simulink model "mrefrobotarm_modified_previous_y_previous_u_previous_ref_pert_2"  (R2018b)
settings: Solver=FixedStepAuto  StartTime=0.0  StopTime=60  RelTol=1e-3  AbsTol=1e-6
undefined symbols (not defined in the file or in its folder): cc, options
libraries: neural x858, simulink x1
(part 10 of 32)

== system mrefrobotarm_modified_previous_y_previous_u_previous_ref_pert_2/m=0 sd=0 original/Layer 3/Delays 1 ==
  "p{3}" : Inport  PortDimensions=30
      mask Display: e = 0.06;c1 = [120 230 180]/255;c2 = ([120 230 180]+0)/(256+128);c3 = ([120 230 180]+128)/(256+128);patch([0 1 1 0],[0 0 1 1],c1);patch([0 1 1 1-e 1-e 0+e],[0 0 1 1-e 0+e 0+e],c2);patch([0 0 1 1-e 0+e 0+e],[0 1 1 1-e 1-e 0+e],c3);plot([0 1 1 0 0],[0 0 1 1 0]);
  mux : Mux  Inputs=1
      mask Display: e = 0.06;c1 = [120 150 230]/255;c2 = ([120 150 230]+0)/383;c3 = ([120 150 230]+128)/383;patch([0 1 1 0],[0 0 1 1],c1);patch([0 1 1 1-e 1-e 0+e],[0 0 1 1-e 0+e 0+e],c2);patch([0 0 1 1-e 0+e 0+e],[0 1 1 1-e 1-e 0+e],c3);plot([0 1 1 0 0],[0 0 1 1 0]);disp('Mux')
  "pd{3,2}" : Outport
      mask Display: e = 0.06;c1 = [120 230 180]/255;c2 = ([120 230 180]+0)/(256+128);c3 = ([120 230 180]+128)/(256+128);patch([0 1 1 0],[0 0 1 1],c1);patch([0 1 1 1-e 1-e 0+e],[0 0 1 1-e 0+e 0+e],c2);patch([0 0 1 1-e 0+e 0+e],[0 1 1 1-e 1-e 0+e],c3);plot([0 1 1 0 0],[0 0 1 1 0]);
  wires:
  "p{3}"/1 -> mux/1
  mux/1 -> "pd{3,2}"/1

== system mrefrobotarm_modified_previous_y_previous_u_previous_ref_pert_2/m=0 sd=0 original/Layer 3/LW{3,2} ==
  "ad{3,2}" : Inport  PortDimensions=30
      mask Display: e = 0.06;c1 = [120 230 180]/255;c2 = ([120 230 180]+0)/(256+128);c3 = ([120 230 180]+128)/(256+128);patch([0 1 1 0],[0 0 1 1],c1);patch([0 1 1 1-e 1-e 0+e],[0 0 1 1-e 0+e 0+e],c2);patch([0 0 1 1-e 0+e 0+e],[0 1 1 1-e 1-e 0+e],c3);plot([0 1 1 0 0],[0 0 1 1 0]);
  "IW{3,2}(1,:)'" : Constant  Value=[0.17482246150930424999359047433244995772838592529296875;0.55622207112490962277462358542834408581256866455078125;0.0031372872160854207122804293561557642533443868160247802734375;-0.168108405397883908793943419368588365614414215087890625;0.05837691976433061202822472068874049000442028045654296875;-0.402959678570381563122992929493193514645099639892578125;-0.167155303188543158388057463525910861790180206298828125;-0.1338968343609756583845182831282727420330047607421875;0.14686670623474251673457047218107618391513824462890625;0.01157271158637744427888360831957470509223639965057373046875;-0.1531146663300509136451665881395456381142139434814453125;0.0190428533611202814579410613760046544484794139862060546875;-0.2039279411341271275315278899142867885529994964599609375;-0.003914288286597765627317091485792843741364777088165283203125;-0.2328617323239242919985514390646130777895450592041015625;0.1159952622429807345127983353449963033199310302734375;0.462684207486491916316850847579189576208591461181640625;-0.01074998441387134580360385172070891712792217731475830078125;-0.464908519270919862176327796987607143819332122802734375;0.098111452853946179430977281299419701099395751953125;0.00777207254254363121004356429466497502289712429046630859375;-0.1946466427188742187581738107837736606597900390625;0.01549753182636756827783575118928638403303921222686767578125;-0.0263655234629284855596420555912118288688361644744873046875;0.11790973762661406676333086807062500156462192535400390625;0.001769238327251491764424695674051690730266273021697998046875;-0.00594124961309642173057365965860299183987081050872802734375;-0.452866633892114067716505587668507359921932220458984375;-0.15777748494897725350938344490714371204376220703125;-0.57998766696437631384952737789717502892017364501953125]
      mask Display: e = 0.06;c1 = [120 150 230]/255;c2 = ([120 150 230]+0)/383;c3 = ([120 150 230]+128)/383;patch([0 1 1 0],[0 0 1 1],c1);patch([0 1 1 1-e 1-e 0+e],[0 0 1 1-e 0+e 0+e],c2);patch([0 0 1 1-e 0+e 0+e],[0 1 1 1-e 1-e 0+e],c3);plot([0 1 1 0 0],[0 0 1 1 0]);disp('weights');
  Mux : Mux  Inputs=1
      mask Display: e = 0.06;c1 = [120 150 230]/255;c2 = ([120 150 230]+0)/383;c3 = ([120 150 230]+128)/383;patch([0 1 1 0],[0 0 1 1],c1);patch([0 1 1 1-e 1-e 0+e],[0 0 1 1-e 0+e 0+e],c2);patch([0 0 1 1-e 0+e 0+e],[0 1 1 1-e 1-e 0+e],c3);plot([0 1 1 0 0],[0 0 1 1 0]);disp('Mux');
  dotprod1 : neural/Weight Functions/dotprod
  "lz{3,2}" : Outport
      mask Display: e = 0.06;c1 = [120 230 180]/255;c2 = ([120 230 180]+0)/(256+128);c3 = ([120 230 180]+128)/(256+128);patch([0 1 1 0],[0 0 1 1],c1);patch([0 1 1 1-e 1-e 0+e],[0 0 1 1-e 0+e 0+e],c2);patch([0 0 1 1-e 0+e 0+e],[0 1 1 1-e 1-e 0+e],c3);plot([0 1 1 0 0],[0 0 1 1 0]);
  wires:
  "IW{3,2}(1,:)'"/1 -> dotprod1/1
  "ad{3,2}"/1 -> dotprod1/2
  dotprod1/1 -> Mux/1
  Mux/1 -> "lz{3,2}"/1

== system mrefrobotarm_modified_previous_y_previous_u_previous_ref_pert_2/m=0 sd=0.001/Layer 1/Delays 1 ==
  "p{1}" : Inport  PortDimensions=10
      mask Display: e = 0.06;c1 = [120 230 180]/255;c2 = ([120 230 180]+0)/(256+128);c3 = ([120 230 180]+128)/(256+128);patch([0 1 1 0],[0 0 1 1],c1);patch([0 1 1 1-e 1-e 0+e],[0 0 1 1-e 0+e 0+e],c2);patch([0 0 1 1-e 0+e 0+e],[0 1 1 1-e 1-e 0+e],c3);plot([0 1 1 0 0],[0 0 1 1 0]);
  mux : Mux  Inputs=1
      mask Display: e = 0.06;c1 = [120 150 230]/255;c2 = ([120 150 230]+0)/383;c3 = ([120 150 230]+128)/383;patch([0 1 1 0],[0 0 1 1],c1);patch([0 1 1 1-e 1-e 0+e],[0 0 1 1-e 0+e 0+e],c2);patch([0 0 1 1-e 0+e 0+e],[0 1 1 1-e 1-e 0+e],c3);plot([0 1 1 0 0],[0 0 1 1 0]);disp('Mux')
  "pd{1,1}" : Outport
      mask Display: e = 0.06;c1 = [120 230 180]/255;c2 = ([120 230 180]+0)/(256+128);c3 = ([120 230 180]+128)/(256+128);patch([0 1 1 0],[0 0 1 1],c1);patch([0 1 1 1-e 1-e 0+e],[0 0 1 1-e 0+e 0+e],c2);patch([0 0 1 1-e 0+e 0+e],[0 1 1 1-e 1-e 0+e],c3);plot([0 1 1 0 0],[0 0 1 1 0]);
  wires:
  "p{1}"/1 -> mux/1
  mux/1 -> "pd{1,1}"/1

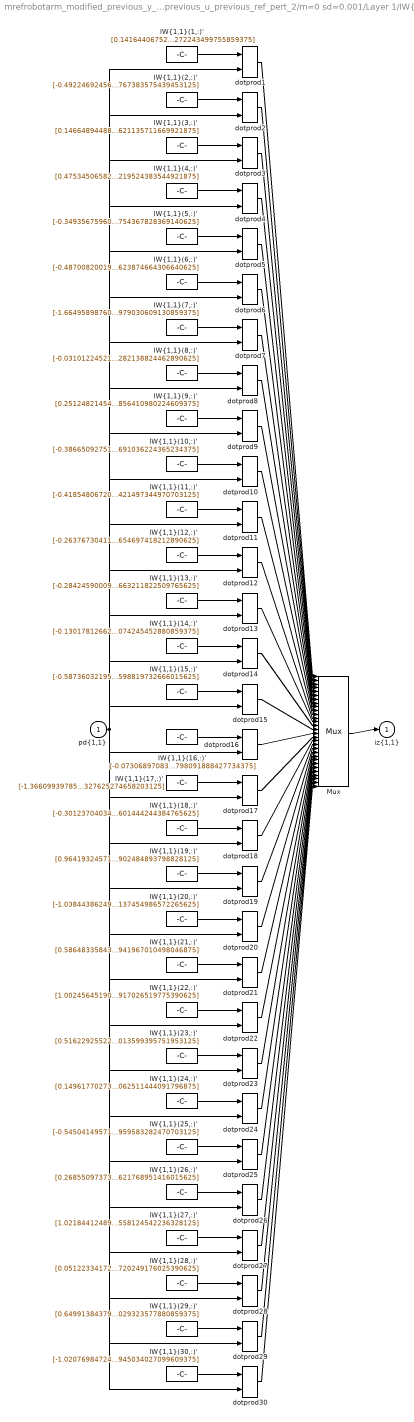
== system mrefrobotarm_modified_previous_y_previous_u_previous_ref_pert_2/m=0 sd=0.001/Layer 1/IW{1,1} ==
  "pd{1,1}" : Inport  PortDimensions=10
      mask Display: e = 0.06;c1 = [120 230 180]/255;c2 = ([120 230 180]+0)/(256+128);c3 = ([120 230 180]+128)/(256+128);patch([0 1 1 0],[0 0 1 1],c1);patch([0 1 1 1-e 1-e 0+e],[0 0 1 1-e 0+e 0+e],c2);patch([0 0 1 1-e 0+e 0+e],[0 1 1 1-e 1-e 0+e],c3);plot([0 1 1 0 0],[0 0 1 1 0]);
  "IW{1,1}(1,:)'" : Constant  Value=[0.141644067527063766132044975165626965463161468505859375;-0.040811020431186666168610344129774603061378002166748046875;-0.312974436634471164797588471628841944038867950439453125;0.04886853485988666701000937564458581618964672088623046875;-0.82641893263483934273239128742716275155544281005859375;-0.91587297277856272170737383930827490985393524169921875;0.67313210047715543726809528379817493259906768798828125;-0.039377277910727627452391885753968381322920322418212890625;-1.2808123988443942398163244433817453682422637939453125;-1.19270082118834519491201717755757272243499755859375]
      mask Display: e = 0.06;c1 = [120 150 230]/255;c2 = ([120 150 230]+0)/383;c3 = ([120 150 230]+128)/383;patch([0 1 1 0],[0 0 1 1],c1);patch([0 1 1 1-e 1-e 0+e],[0 0 1 1-e 0+e 0+e],c2);patch([0 0 1 1-e 0+e 0+e],[0 1 1 1-e 1-e 0+e],c3);plot([0 1 1 0 0],[0 0 1 1 0]);disp('Weights');
  "IW{1,1}(10,:)'" : Constant  Value=[-0.38665092751456509034824193804524838924407958984375;0.06410981472709277595445342967650503851473331451416015625;0.11657362993113169757908309520644252188503742218017578125;0.034769749880571333700007841116530471481382846832275390625;-0.2113731343708413479287600011957692913711071014404296875;1.3959509118760367041289782719104550778865814208984375;-1.3344611781825508334264895893284119665622711181640625;-0.26325521537912710545725758493063040077686309814453125;1.11568339513819214658951750607229769229888916015625;0.285147448344198417569117509628995321691036224365234375]
      mask Display: e = 0.06;c1 = [120 150 230]/255;c2 = ([120 150 230]+0)/383;c3 = ([120 150 230]+128)/383;patch([0 1 1 0],[0 0 1 1],c1);patch([0 1 1 1-e 1-e 0+e],[0 0 1 1-e 0+e 0+e],c2);patch([0 0 1 1-e 0+e 0+e],[0 1 1 1-e 1-e 0+e],c3);plot([0 1 1 0 0],[0 0 1 1 0]);disp('Weights');
  "IW{1,1}(11,:)'" : Constant  Value=[-0.4185480672053982775793201653868891298770904541015625;-0.1705980694049138157719625041863764636218547821044921875;-0.0190899797350324341993488275193158187903463840484619140625;-0.327569152910229366426619890262372791767120361328125;0.1274098816431911418423084114692755974829196929931640625;-1.9161340172549110594246712935273535549640655517578125;0.05443650875980780845520001776094431988894939422607421875;0.32968385223698126740288216751650907099246978759765625;-0.98609685726316964604620807222090661525726318359375;-1.012171418694518099101742336642928421497344970703125]
      mask Display: e = 0.06;c1 = [120 150 230]/255;c2 = ([120 150 230]+0)/383;c3 = ([120 150 230]+128)/383;patch([0 1 1 0],[0 0 1 1],c1);patch([0 1 1 1-e 1-e 0+e],[0 0 1 1-e 0+e 0+e],c2);patch([0 0 1 1-e 0+e 0+e],[0 1 1 1-e 1-e 0+e],c3);plot([0 1 1 0 0],[0 0 1 1 0]);disp('Weights');
  "IW{1,1}(12,:)'" : Constant  Value=[-0.263767304113963263478837006914545781910419464111328125;-0.629903348227637049916438627406023442745208740234375;0.7293914306477302655906669315299950540065765380859375;0.1405283307055230357374142613480216823518276214599609375;1.7781482645602564307552029276848770678043365478515625;-2.97153163801516040365413573454134166240692138671875;0.443336274156811371849329361793934367597103118896484375;0.55612212810498140580506287733442150056362152099609375;-0.1887978911441915153002213401123299263417720794677734375;-0.55133598654912996384069856503629125654697418212890625]
      mask Display: e = 0.06;c1 = [120 150 230]/255;c2 = ([120 150 230]+0)/383;c3 = ([120 150 230]+128)/383;patch([0 1 1 0],[0 0 1 1],c1);patch([0 1 1 1-e 1-e 0+e],[0 0 1 1-e 0+e 0+e],c2);patch([0 0 1 1-e 0+e 0+e],[0 1 1 1-e 1-e 0+e],c3);plot([0 1 1 0 0],[0 0 1 1 0]);disp('Weights');
  "IW{1,1}(13,:)'" : Constant  Value=[-0.2842459000975889882312230838579125702381134033203125;-0.07040272701257387077955485210623010061681270599365234375;-0.279039840893809010236026324491831474006175994873046875;-0.89305639600684505463590312501764856278896331787109375;3.341208886966132052265265883761458098888397216796875;-1.98213319967933188081588014028966426849365234375;-0.90166622936895013395997011684812605381011962890625;0.2060321618557637013413597060207393951714038848876953125;0.00677792762518984910624642026277797413058578968048095703125;0.7006967694845107619272539523080922663211822509765625]
      mask Display: e = 0.06;c1 = [120 150 230]/255;c2 = ([120 150 230]+0)/383;c3 = ([120 150 230]+128)/383;patch([0 1 1 0],[0 0 1 1],c1);patch([0 1 1 1-e 1-e 0+e],[0 0 1 1-e 0+e 0+e],c2);patch([0 0 1 1-e 0+e 0+e],[0 1 1 1-e 1-e 0+e],c3);plot([0 1 1 0 0],[0 0 1 1 0]);disp('Weights');
  "IW{1,1}(14,:)'" : Constant  Value=[-0.130178126624194090421582359340391121804714202880859375;-0.57366570129351235340919856753316707909107208251953125;0.339047467618743325612484795783529989421367645263671875;0.09356817756562685328702855258597992360591888427734375;-2.342341044490604762273733285837806761264801025390625;0.73263251994819456047736139225889928638935089111328125;-1.0945043994785914609479959835880436003208160400390625;0.36014660154459676721927507969667203724384307861328125;0.08590539675617943349283933685001102276146411895751953125;0.294060428112707439307627055313787423074245452880859375]
      mask Display: e = 0.06;c1 = [120 150 230]/255;c2 = ([120 150 230]+0)/383;c3 = ([120 150 230]+128)/383;patch([0 1 1 0],[0 0 1 1],c1);patch([0 1 1 1-e 1-e 0+e],[0 0 1 1-e 0+e 0+e],c2);patch([0 0 1 1-e 0+e 0+e],[0 1 1 1-e 1-e 0+e],c3);plot([0 1 1 0 0],[0 0 1 1 0]);disp('Weights');
  "IW{1,1}(15,:)'" : Constant  Value=[-0.58736032195968690405862844272633083164691925048828125;-0.97694049420584827547742179376655258238315582275390625;0.445085876738007313324629876660765148699283599853515625;-0.81400813268761462726530453437590040266513824462890625;1.0180878938153157253765357381780631840229034423828125;3.209784057241337418275861637084744870662689208984375;-3.79904217491637385961666950606741011142730712890625;-1.092793036625193447974879745743237435817718505859375;0.14930752660064150472152277870918624103069305419921875;0.05185259448477598509530395176625461317598819732666015625]
      mask Display: e = 0.06;c1 = [120 150 230]/255;c2 = ([120 150 230]+0)/383;c3 = ([120 150 230]+128)/383;patch([0 1 1 0],[0 0 1 1],c1);patch([0 1 1 1-e 1-e 0+e],[0 0 1 1-e 0+e 0+e],c2);patch([0 0 1 1-e 0+e 0+e],[0 1 1 1-e 1-e 0+e],c3);plot([0 1 1 0 0],[0 0 1 1 0]);disp('Weights');
  "IW{1,1}(16,:)'" : Constant  Value=[-0.07306897083321206576300710366922430694103240966796875;1.336326295485117388039952857070602476596832275390625;-0.7720355294134737533795487252064049243927001953125;-0.0139085855546657900794205175998285994865000247955322265625;-0.0206566869740357310358813691664181533269584178924560546875;-1.71478968915085960844635337707586586475372314453125;1.2257029083013410986069402497378177940845489501953125;-0.09002770556177196181746325009953579865396022796630859375;0.11941733786638293601800597798501257784664630889892578125;-0.90605832310140266283582377582206390798091888427734375]
      mask Display: e = 0.06;c1 = [120 150 230]/255;c2 = ([120 150 230]+0)/383;c3 = ([120 150 230]+128)/383;patch([0 1 1 0],[0 0 1 1],c1);patch([0 1 1 1-e 1-e 0+e],[0 0 1 1-e 0+e 0+e],c2);patch([0 0 1 1-e 0+e 0+e],[0 1 1 1-e 1-e 0+e],c3);plot([0 1 1 0 0],[0 0 1 1 0]);disp('Weights');
  "IW{1,1}(17,:)'" : Constant  Value=[-1.3660993978584310415413938244455493986606597900390625;0.447368239870595318929957784348516725003719329833984375;-0.3151903130669932995289173049968667328357696533203125;0.5490665053490355607124229209148325026035308837890625;-1.3878202169631757012524531091912649571895599365234375;0.8786192170572351134438804365345276892185211181640625;1.262628679383082985765440753311850130558013916015625;0.058805307505513125521101613912833272479474544525146484375;-1.1570038544094110033455535813118331134319305419921875;-0.5372653883201519153800518324715085327625274658203125]
      mask Display: e = 0.06;c1 = [120 150 230]/255;c2 = ([120 150 230]+0)/383;c3 = ([120 150 230]+128)/383;patch([0 1 1 0],[0 0 1 1],c1);patch([0 1 1 1-e 1-e 0+e],[0 0 1 1-e 0+e 0+e],c2);patch([0 0 1 1-e 0+e 0+e],[0 1 1 1-e 1-e 0+e],c3);plot([0 1 1 0 0],[0 0 1 1 0]);disp('Weights');
  "IW{1,1}(18,:)'" : Constant  Value=[-0.30123704034130949214187467077863402664661407470703125;-0.9826928772233014530712580381077714264392852783203125;0.458807999760197537941763812341378070414066314697265625;-0.40943441195293439616165187544538639485836029052734375;3.18222944124208506622153436182998120784759521484375;-3.59620492037495775861088986857794225215911865234375;-0.65381206466542629573979183987830765545368194580078125;-0.382872313537668429450633311716956086456775665283203125;-0.2265333512022854878242839049562462605535984039306640625;-0.29065348270207513881047134418622590601444244384765625]
      mask Display: e = 0.06;c1 = [120 150 230]/255;c2 = ([120 150 230]+0)/383;c3 = ([120 150 230]+128)/383;patch([0 1 1 0],[0 0 1 1],c1);patch([0 1 1 1-e 1-e 0+e],[0 0 1 1-e 0+e 0+e],c2);patch([0 0 1 1-e 0+e 0+e],[0 1 1 1-e 1-e 0+e],c3);plot([0 1 1 0 0],[0 0 1 1 0]);disp('Weights');
  "IW{1,1}(19,:)'" : Constant  Value=[0.96419324571240772048241751690511591732501983642578125;-1.3244739761707375880206427609664388000965118408203125;0.71099355709791201007874406059272587299346923828125;0.58689421989973367121962155579240061342716217041015625;0.334618188188679110961487594977370463311672210693359375;0.84737434997447624862587645111489109694957733154296875;-1.6900909118182274593067404566681943833827972412109375;0.88269403343754671009691037397715263068675994873046875;1.8107083934901881949741664357134141027927398681640625;1.2484881688190185844433699458022601902484893798828125]
      mask Display: e = 0.06;c1 = [120 150 230]/255;c2 = ([120 150 230]+0)/383;c3 = ([120 150 230]+128)/383;patch([0 1 1 0],[0 0 1 1],c1);patch([0 1 1 1-e 1-e 0+e],[0 0 1 1-e 0+e 0+e],c2);patch([0 0 1 1-e 0+e 0+e],[0 1 1 1-e 1-e 0+e],c3);plot([0 1 1 0 0],[0 0 1 1 0]);disp('Weights');
  "IW{1,1}(2,:)'" : Constant  Value=[-0.4922469245624248035397840794757939875125885009765625;1.5643186757990494850645291080581955611705780029296875;-0.53292067555930422440013671803171746432781219482421875;-0.9036943745991286025542876814142800867557525634765625;0.91836790007748325681546930354670621454715728759765625;0.797764212943369965813644739682786166667938232421875;-0.8263507117606658791686413678689859807491302490234375;-1.0307819223642396000428789193392731249332427978515625;0.1122702889794594260930438167633838020265102386474609375;-0.266823200656654269113943200864014215767383575439453125]
      mask Display: e = 0.06;c1 = [120 150 230]/255;c2 = ([120 150 230]+0)/383;c3 = ([120 150 230]+128)/383;patch([0 1 1 0],[0 0 1 1],c1);patch([0 1 1 1-e 1-e 0+e],[0 0 1 1-e 0+e 0+e],c2);patch([0 0 1 1-e 0+e 0+e],[0 1 1 1-e 1-e 0+e],c3);plot([0 1 1 0 0],[0 0 1 1 0]);disp('Weights');
  "IW{1,1}(20,:)'" : Constant  Value=[-1.0384438624947509577367554811644367873668670654296875;-0.6857372712514451240650714680668897926807403564453125;1.1134932996860460452381857976433821022510528564453125;0.231336892081496936501849859268986620008945465087890625;0.06468854520925941542497383807130972854793071746826171875;1.6504256276818247695103991645737551152706146240234375;-1.8766143549175211546753416769206523895263671875;0.50621961059078068867478350512101314961910247802734375;1.0039049993566824259261238694307394325733184814453125;0.2142061738710933360696486715823994018137454986572265625]
      mask Display: e = 0.06;c1 = [120 150 230]/255;c2 = ([120 150 230]+0)/383;c3 = ([120 150 230]+128)/383;patch([0 1 1 0],[0 0 1 1],c1);patch([0 1 1 1-e 1-e 0+e],[0 0 1 1-e 0+e 0+e],c2);patch([0 0 1 1-e 0+e 0+e],[0 1 1 1-e 1-e 0+e],c3);plot([0 1 1 0 0],[0 0 1 1 0]);disp('Weights');
  "IW{1,1}(21,:)'" : Constant  Value=[0.586483358430462065058463849709369242191314697265625;0.9441412228798997663403724800446070730686187744140625;-0.179250313262965033089813005062751471996307373046875;0.1543817479365020839399136320935213007032871246337890625;1.7772297766169808941327801221632398664951324462890625;-0.185911672646862646818277653437689878046512603759765625;0.309147974345889864355996223821421153843402862548828125;0.367275542109159525150374747681780718266963958740234375;-0.29157553027840032999762343024485744535923004150390625;-0.491040472831766106054374176892451941967010498046875]
      mask Display: e = 0.06;c1 = [120 150 230]/255;c2 = ([120 150 230]+0)/383;c3 = ([120 150 230]+128)/383;patch([0 1 1 0],[0 0 1 1],c1);patch([0 1 1 1-e 1-e 0+e],[0 0 1 1-e 0+e 0+e],c2);patch([0 0 1 1-e 0+e 0+e],[0 1 1 1-e 1-e 0+e],c3);plot([0 1 1 0 0],[0 0 1 1 0]);disp('Weights');
  "IW{1,1}(22,:)'" : Constant  Value=[1.0024564519061993639326146876555867493152618408203125;1.0876807186297920981843390109133906662464141845703125;-1.1612223118807827315634995102300308644771575927734375;-0.1525238500425340759658610068072448484599590301513671875;-1.2099756469466800279377594051766209304332733154296875;1.56156892463482765975868460373021662235260009765625;-0.744987882196795681011280976235866546630859375;-0.553211696967941701785775876487605273723602294921875;-0.06571733242353128279233942521386779844760894775390625;-0.50385468889715756546365810208953917026519775390625]
      mask Display: e = 0.06;c1 = [120 150 230]/255;c2 = ([120 150 230]+0)/383;c3 = ([120 150 230]+128)/383;patch([0 1 1 0],[0 0 1 1],c1);patch([0 1 1 1-e 1-e 0+e],[0 0 1 1-e 0+e 0+e],c2);patch([0 0 1 1-e 0+e 0+e],[0 1 1 1-e 1-e 0+e],c3);plot([0 1 1 0 0],[0 0 1 1 0]);disp('Weights');
  "IW{1,1}(23,:)'" : Constant  Value=[0.5162292552287526259391370331286452710628509521484375;0.2402443418112102102579541451632394455373287200927734375;0.357558744801976857718983637823839671909809112548828125;0.55513687772271358422671028165495954453945159912109375;0.33837883366245069538535972242243587970733642578125;-0.051111627444114231255678504339812207035720348358154296875;0.89939482304013040891987884606351144611835479736328125;-0.77119186462660849201711243949830532073974609375;-0.2217442499175407422118411204792209900915622711181640625;0.2276515633989102671552728907045093365013599395751953125]
      mask Display: e = 0.06;c1 = [120 150 230]/255;c2 = ([120 150 230]+0)/383;c3 = ([120 150 230]+128)/383;patch([0 1 1 0],[0 0 1 1],c1);patch([0 1 1 1-e 1-e 0+e],[0 0 1 1-e 0+e 0+e],c2);patch([0 0 1 1-e 0+e 0+e],[0 1 1 1-e 1-e 0+e],c3);plot([0 1 1 0 0],[0 0 1 1 0]);disp('Weights');
  "IW{1,1}(24,:)'" : Constant  Value=[0.1496177027304214368630397302695200778543949127197265625;0.36158960674317264238908364859526045620441436767578125;-0.25587623983823803985870881660957820713520050048828125;0.33843273918136163036507468859781511127948760986328125;-0.6329021269091421597607904914184473454952239990234375;0.87679403200243111182743405151995830237865447998046875;0.0925381072310929309043814328106236644089221954345703125;0.73329866113122388338041446331772021949291229248046875;-0.1551914224368062533709888839439372532069683074951171875;1.0203455540178072435963940733927302062511444091796875]
      mask Display: e = 0.06;c1 = [120 150 230]/255;c2 = ([120 150 230]+0)/383;c3 = ([120 150 230]+128)/383;patch([0 1 1 0],[0 0 1 1],c1);patch([0 1 1 1-e 1-e 0+e],[0 0 1 1-e 0+e 0+e],c2);patch([0 0 1 1-e 0+e 0+e],[0 1 1 1-e 1-e 0+e],c3);plot([0 1 1 0 0],[0 0 1 1 0]);disp('Weights');
  "IW{1,1}(25,:)'" : Constant  Value=[-0.545041495714835289021493736072443425655364990234375;1.240168195401757156304256568546406924724578857421875;-0.6762745807714889423323256778530776500701904296875;0.029711242629012334093285829794695018790662288665771484375;-0.272618060906240577967452054508612491190433502197265625;-0.1782320475966485684438112002681009471416473388671875;0.830680966188705127706271014176309108734130859375;-0.64531493370986370283759470112272538244724273681640625;-0.297498345299267830110778731977916322648525238037109375;-1.0164389843838332883052544275415129959583282470703125]
      mask Display: e = 0.06;c1 = [120 150 230]/255;c2 = ([120 150 230]+0)/383;c3 = ([120 150 230]+128)/383;patch([0 1 1 0],[0 0 1 1],c1);patch([0 1 1 1-e 1-e 0+e],[0 0 1 1-e 0+e 0+e],c2);patch([0 0 1 1-e 0+e 0+e],[0 1 1 1-e 1-e 0+e],c3);plot([0 1 1 0 0],[0 0 1 1 0]);disp('Weights');
  "IW{1,1}(26,:)'" : Constant  Value=[0.268550973733946263255489839139045216143131256103515625;-0.6727690633528127239770810774643905460834503173828125;0.278948136101189458901927764600259251892566680908203125;0.57936309348644121630655945409671403467655181884765625;1.163501734027301726115410929196514189243316650390625;-2.368390781074349860091388109140098094940185546875;0.62965079555685132817188787157647311687469482421875;0.74588303521310839183655616579926572740077972412109375;0.91722762005284075303990221073036082088947296142578125;0.42716514786234738298986712834448553621768951416015625]
      mask Display: e = 0.06;c1 = [120 150 230]/255;c2 = ([120 150 230]+0)/383;c3 = ([120 150 230]+128)/383;patch([0 1 1 0],[0 0 1 1],c1);patch([0 1 1 1-e 1-e 0+e],[0 0 1 1-e 0+e 0+e],c2);patch([0 0 1 1-e 0+e 0+e],[0 1 1 1-e 1-e 0+e],c3);plot([0 1 1 0 0],[0 0 1 1 0]);disp('Weights');
  "IW{1,1}(27,:)'" : Constant  Value=[1.021844124898213745922248563147149980068206787109375;0.11691700672593856313863369678074377588927745819091796875;-0.442221536021734140664563028622069396078586578369140625;-0.5381148934229027513964638274046592414379119873046875;0.132566187839600557740737940548569895327091217041015625;0.423366665945351494659831814715289510786533355712890625;0.96024082132894517105370368881267495453357696533203125;-1.1841214698932844839873723685741424560546875;-1.1472381571134058209082695611868984997272491455078125;0.44719708863346341320976762290229089558124542236328125]
      mask Display: e = 0.06;c1 = [120 150 230]/255;c2 = ([120 150 230]+0)/383;c3 = ([120 150 230]+128)/383;patch([0 1 1 0],[0 0 1 1],c1);patch([0 1 1 1-e 1-e 0+e],[0 0 1 1-e 0+e 0+e],c2);patch([0 0 1 1-e 0+e 0+e],[0 1 1 1-e 1-e 0+e],c3);plot([0 1 1 0 0],[0 0 1 1 0]);disp('Weights');
  "IW{1,1}(28,:)'" : Constant  Value=[0.051223341726610381596795917857889435254037380218505859375;-0.48294213843193956048338577602407895028591156005859375;0.5299034774992252838643480572500266134738922119140625;-0.0181855933119925150531770441375556401908397674560546875;-0.55600820600733380505431568963103927671909332275390625;-0.37056590490196505971454143946175463497638702392578125;0.52603994879513482629818099667318165302276611328125;0.480248998928426040766481719401781447231769561767578125;-1.199673965797023900137219243333674967288970947265625;0.58579556186806147621837226324714720249176025390625]
      mask Display: e = 0.06;c1 = [120 150 230]/255;c2 = ([120 150 230]+0)/383;c3 = ([120 150 230]+128)/383;patch([0 1 1 0],[0 0 1 1],c1);patch([0 1 1 1-e 1-e 0+e],[0 0 1 1-e 0+e 0+e],c2);patch([0 0 1 1-e 0+e 0+e],[0 1 1 1-e 1-e 0+e],c3);plot([0 1 1 0 0],[0 0 1 1 0]);disp('Weights');
  "IW{1,1}(29,:)'" : Constant  Value=[0.6499138437995473083219621912576258182525634765625;0.042631963332267541755271622605505399405956268310546875;-0.029805698786010074996521979073804686777293682098388671875;-1.1046748933898744571280303716775961220264434814453125;0.09622980043175637099306385380259598605334758758544921875;0.94807641538273823567095632824930362403392791748046875;-1.1658660208503028865578698969329707324504852294921875;-0.5163805715088496395281936202081851661205291748046875;-1.3947968786633866411506232907413505017757415771484375;-0.460957399153350377840610008206567727029323577880859375]
      mask Display: e = 0.06;c1 = [120 150 230]/255;c2 = ([120 150 230]+0)/383;c3 = ([120 150 230]+128)/383;patch([0 1 1 0],[0 0 1 1],c1);patch([0 1 1 1-e 1-e 0+e],[0 0 1 1-e 0+e 0+e],c2);patch([0 0 1 1-e 0+e 0+e],[0 1 1 1-e 1-e 0+e],c3);plot([0 1 1 0 0],[0 0 1 1 0]);disp('Weights');
  "IW{1,1}(3,:)'" : Constant  Value=[0.1466489448839114750899881300938432104885578155517578125;0.285419862592237338905221122331568039953708648681640625;-0.1418549021593980830058256970005459152162075042724609375;-1.086697246559418683631292878999374806880950927734375;1.140461418590430042740990757010877132415771484375;0.95861538254347766763174831794458441436290740966796875;-1.679881474998133672471567479078657925128936767578125;-0.7540743679006014499321963739930652081966400146484375;-0.369600199590198130739082671425421722233295440673828125;0.77087480543652453501834997950936667621135711669921875]
      mask Display: e = 0.06;c1 = [120 150 230]/255;c2 = ([120 150 230]+0)/383;c3 = ([120 150 230]+128)/383;patch([0 1 1 0],[0 0 1 1],c1);patch([0 1 1 1-e 1-e 0+e],[0 0 1 1-e 0+e 0+e],c2);patch([0 0 1 1-e 0+e 0+e],[0 1 1 1-e 1-e 0+e],c3);plot([0 1 1 0 0],[0 0 1 1 0]);disp('Weights');
  "IW{1,1}(30,:)'" : Constant  Value=[-1.02076984724676744775706538348458707332611083984375;0.9073144019396879311756265451549552381038665771484375;0.316184113431888125234081599046476185321807861328125;-0.903751501440513305141166711109690368175506591796875;-0.05788614232744225540638893789946450851857662200927734375;0.048205678285076040967549459992369520477950572967529296875;0.71689634449991557207937376006157137453556060791015625;-0.79289973555986736908351986130583100020885467529296875;-0.6839655563035267338278799797990359365940093994140625;-0.359762819657480914514735559350810945034027099609375]
      mask Display: e = 0.06;c1 = [120 150 230]/255;c2 = ([120 150 230]+0)/383;c3 = ([120 150 230]+128)/383;patch([0 1 1 0],[0 0 1 1],c1);patch([0 1 1 1-e 1-e 0+e],[0 0 1 1-e 0+e 0+e],c2);patch([0 0 1 1-e 0+e 0+e],[0 1 1 1-e 1-e 0+e],c3);plot([0 1 1 0 0],[0 0 1 1 0]);disp('Weights');
  "IW{1,1}(4,:)'" : Constant  Value=[0.47534506582431690357992692952393554151058197021484375;0.103864955204604758609576720118639059364795684814453125;-0.6018352797899713113594089008984155952930450439453125;0.833874671666058109309460633085109293460845947265625;-0.2013249670959192660912862038458115421235561370849609375;-0.98652233416476764471525484623271040618419647216796875;-0.345427889677839716764395916470675729215145111083984375;0.77885611910695351500777405817643739283084869384765625;-0.82463653780805679094356719360803253948688507080078125;0.49075841745674331217941244176472537219524383544921875]
      mask Display: e = 0.06;c1 = [120 150 230]/255;c2 = ([120 150 230]+0)/383;c3 = ([120 150 230]+128)/383;patch([0 1 1 0],[0 0 1 1],c1);patch([0 1 1 1-e 1-e 0+e],[0 0 1 1-e 0+e 0+e],c2);patch([0 0 1 1-e 0+e 0+e],[0 1 1 1-e 1-e 0+e],c3);plot([0 1 1 0 0],[0 0 1 1 0]);disp('Weights');
  "IW{1,1}(5,:)'" : Constant  Value=[-0.34935675960055523336933447353658266365528106689453125;0.9502024089757734603978178711258806288242340087890625;-0.50651233603255285675714958415483124554157257080078125;-0.1872869812992668803186546711003757081925868988037109375;0.89708024976171107933708981363452039659023284912109375;-1.54980510833009343940602775546722114086151123046875;0.973865924945797711842487842659465968608856201171875;-0.088119244574121236013297675526700913906097412109375;-0.852212361268162243987944748369045555591583251953125;-0.9897759161133239391716642785468138754367828369140625]
      mask Display: e = 0.06;c1 = [120 150 230]/255;c2 = ([120 150 230]+0)/383;c3 = ([120 150 230]+128)/383;patch([0 1 1 0],[0 0 1 1],c1);patch([0 1 1 1-e 1-e 0+e],[0 0 1 1-e 0+e 0+e],c2);patch([0 0 1 1-e 0+e 0+e],[0 1 1 1-e 1-e 0+e],c3);plot([0 1 1 0 0],[0 0 1 1 0]);disp('Weights');
  "IW{1,1}(6,:)'" : Constant  Value=[-0.48700820019242219149901984565076418220996856689453125;1.047980410435080056430479089613072574138641357421875;-0.5388041052370147188099736013100482523441314697265625;-0.00795863147971094531119007342567783780395984649658203125;0.2264923942275635371235154025271185673773288726806640625;-0.45564641374523595640511075544054619967937469482421875;0.71433468971979452444287517209886573255062103271484375;-0.3244036494570516904190071727498434484004974365234375;-0.19674821845171430734211526214494369924068450927734375;-0.61675829090089140382957566544064320623874664306640625]
      mask Display: e = 0.06;c1 = [120 150 230]/255;c2 = ([120 150 230]+0)/383;c3 = ([120 150 230]+128)/383;patch([0 1 1 0],[0 0 1 1],c1);patch([0 1 1 1-e 1-e 0+e],[0 0 1 1-e 0+e 0+e],c2);patch([0 0 1 1-e 0+e 0+e],[0 1 1 1-e 1-e 0+e],c3);plot([0 1 1 0 0],[0 0 1 1 0]);disp('Weights');
  "IW{1,1}(7,:)'" : Constant  Value=[-1.6649589876043398017912977593368850648403167724609375;-0.08022311161491572917281445143089513294398784637451171875;0.704989602055255293322488796547986567020416259765625;-0.2320372817282516375581025158680859021842479705810546875;0.293735781702903764323053792395512573421001434326171875;1.102383008051555091100226491107605397701263427734375;0.0272699384329121129189044125951113528572022914886474609375;-0.1802490083694523737012360697917756624519824981689453125;0.68201688025299278539392844322719611227512359619140625;-1.1685126414315119003362042349181137979030609130859375]
      mask Display: e = 0.06;c1 = [120 150 230]/255;c2 = ([120 150 230]+0)/383;c3 = ([120 150 230]+128)/383;patch([0 1 1 0],[0 0 1 1],c1);patch([0 1 1 1-e 1-e 0+e],[0 0 1 1-e 0+e 0+e],c2);patch([0 0 1 1-e 0+e 0+e],[0 1 1 1-e 1-e 0+e],c3);plot([0 1 1 0 0],[0 0 1 1 0]);disp('Weights');
  "IW{1,1}(8,:)'" : Constant  Value=[-0.0310122452179960872431507823421270586550235748291015625;-0.69283103819093405650875183710013516247272491455078125;0.917832482071700983539130902499891817569732666015625;0.26034290904793622178914347387035377323627471923828125;1.8491303137488677155175764710293151438236236572265625;-1.28010485236966697897287303931079804897308349609375;-0.85686933918454510905604593062889762222766876220703125;0.290063752012217346276656826375983655452728271484375;0.976893783547704952496815167251043021678924560546875;0.4078549397232686946068724864744581282138824462890625]
      mask Display: e = 0.06;c1 = [120 150 230]/255;c2 = ([120 150 230]+0)/383;c3 = ([120 150 230]+128)/383;patch([0 1 1 0],[0 0 1 1],c1);patch([0 1 1 1-e 1-e 0+e],[0 0 1 1-e 0+e 0+e],c2);patch([0 0 1 1-e 0+e 0+e],[0 1 1 1-e 1-e 0+e],c3);plot([0 1 1 0 0],[0 0 1 1 0]);disp('Weights');
  "IW{1,1}(9,:)'" : Constant  Value=[0.25124821454878432103186014501261524856090545654296875;-0.211580262050472089896402394515462219715118408203125;0.182973334861581016230758223173324950039386749267578125;-0.08017621098171011373434424740480608306825160980224609375;-0.404551974614447862332866634460515342652797698974609375;1.0485061897571055222755376234999857842922210693359375;-0.48746856605480115565143250933033414185047149658203125;-0.424373078791534463771739638104918412864208221435546875;-0.91920076415423068727506006325711496174335479736328125;-1.09852844034877872303468393511138856410980224609375]
      mask Display: e = 0.06;c1 = [120 150 230]/255;c2 = ([120 150 230]+0)/383;c3 = ([120 150 230]+128)/383;patch([0 1 1 0],[0 0 1 1],c1);patch([0 1 1 1-e 1-e 0+e],[0 0 1 1-e 0+e 0+e],c2);patch([0 0 1 1-e 0+e 0+e],[0 1 1 1-e 1-e 0+e],c3);plot([0 1 1 0 0],[0 0 1 1 0]);disp('Weights');
  Mux : Mux  Inputs=30
      mask Display: e = 0.06;c1 = [120 150 230]/255;c2 = ([120 150 230]+0)/383;c3 = ([120 150 230]+128)/383;patch([0 1 1 0],[0 0 1 1],c1);patch([0 1 1 1-e 1-e 0+e],[0 0 1 1-e 0+e 0+e],c2);patch([0 0 1 1-e 0+e 0+e],[0 1 1 1-e 1-e 0+e],c3);plot([0 1 1 0 0],[0 0 1 1 0]);disp('Mux');
  dotprod{1..30} (30 alike) : neural/Weight Functions/dotprod
  "iz{1,1}" : Outport
      mask Display: e = 0.06;c1 = [120 230 180]/255;c2 = ([120 230 180]+0)/(256+128);c3 = ([120 230 180]+128)/(256+128);patch([0 1 1 0],[0 0 1 1],c1);patch([0 1 1 1-e 1-e 0+e],[0 0 1 1-e 0+e 0+e],c2);patch([0 0 1 1-e 0+e 0+e],[0 1 1 1-e 1-e 0+e],c3);plot([0 1 1 0 0],[0 0 1 1 0]);
  wires:
  "IW{1,1}(1,:)'"/1 -> dotprod1/1
  "pd{1,1}"/1 -> dotprod1/2, dotprod2/2, dotprod3/2, dotprod4/2, dotprod5/2, dotprod6/2, dotprod7/2, dotprod8/2, dotprod9/2, dotprod10/2, dotprod11/2, dotprod12/2, dotprod13/2, dotprod14/2, dotprod15/2, dotprod16/2, dotprod17/2, dotprod18/2, dotprod19/2, dotprod20/2, dotprod21/2, dotprod22/2, dotprod23/2, dotprod24/2, dotprod25/2, dotprod26/2, dotprod27/2, dotprod28/2, dotprod29/2, dotprod30/2
  dotprod1/1 -> Mux/1
  "IW{1,1}(2,:)'"/1 -> dotprod2/1
  dotprod2/1 -> Mux/2
  "IW{1,1}(3,:)'"/1 -> dotprod3/1
  dotprod3/1 -> Mux/3
  "IW{1,1}(4,:)'"/1 -> dotprod4/1
  dotprod4/1 -> Mux/4
  "IW{1,1}(5,:)'"/1 -> dotprod5/1
  dotprod5/1 -> Mux/5
  "IW{1,1}(6,:)'"/1 -> dotprod6/1
  dotprod6/1 -> Mux/6
  "IW{1,1}(7,:)'"/1 -> dotprod7/1
  dotprod7/1 -> Mux/7
  "IW{1,1}(8,:)'"/1 -> dotprod8/1
  dotprod8/1 -> Mux/8
  "IW{1,1}(9,:)'"/1 -> dotprod9/1
  dotprod9/1 -> Mux/9
  "IW{1,1}(10,:)'"/1 -> dotprod10/1
  dotprod10/1 -> Mux/10
  "IW{1,1}(11,:)'"/1 -> dotprod11/1
  dotprod11/1 -> Mux/11
  "IW{1,1}(12,:)'"/1 -> dotprod12/1
  dotprod12/1 -> Mux/12
  "IW{1,1}(13,:)'"/1 -> dotprod13/1
  dotprod13/1 -> Mux/13
  "IW{1,1}(14,:)'"/1 -> dotprod14/1
  dotprod14/1 -> Mux/14
  "IW{1,1}(15,:)'"/1 -> dotprod15/1
  dotprod15/1 -> Mux/15
  "IW{1,1}(16,:)'"/1 -> dotprod16/1
  dotprod16/1 -> Mux/16
  "IW{1,1}(17,:)'"/1 -> dotprod17/1
  dotprod17/1 -> Mux/17
  "IW{1,1}(18,:)'"/1 -> dotprod18/1
  dotprod18/1 -> Mux/18
  "IW{1,1}(19,:)'"/1 -> dotprod19/1
  dotprod19/1 -> Mux/19
  "IW{1,1}(20,:)'"/1 -> dotprod20/1
  dotprod20/1 -> Mux/20
  "IW{1,1}(21,:)'"/1 -> dotprod21/1
  dotprod21/1 -> Mux/21
  "IW{1,1}(22,:)'"/1 -> dotprod22/1
  dotprod22/1 -> Mux/22
  "IW{1,1}(23,:)'"/1 -> dotprod23/1
  dotprod23/1 -> Mux/23
  "IW{1,1}(24,:)'"/1 -> dotprod24/1
  dotprod24/1 -> Mux/24
  "IW{1,1}(25,:)'"/1 -> dotprod25/1
  dotprod25/1 -> Mux/25
  "IW{1,1}(26,:)'"/1 -> dotprod26/1
  dotprod26/1 -> Mux/26
  "IW{1,1}(27,:)'"/1 -> dotprod27/1
  dotprod27/1 -> Mux/27
  "IW{1,1}(28,:)'"/1 -> dotprod28/1
  dotprod28/1 -> Mux/28
  "IW{1,1}(29,:)'"/1 -> dotprod29/1
  dotprod29/1 -> Mux/29
  "IW{1,1}(30,:)'"/1 -> dotprod30/1
  dotprod30/1 -> Mux/30
  Mux/1 -> "iz{1,1}"/1

== system mrefrobotarm_modified_previous_y_previous_u_previous_ref_pert_2/m=0 sd=0.001/Layer 2/Delays 1 ==
  "p{2}" : Inport  PortDimensions=30
      mask Display: e = 0.06;c1 = [120 230 180]/255;c2 = ([120 230 180]+0)/(256+128);c3 = ([120 230 180]+128)/(256+128);patch([0 1 1 0],[0 0 1 1],c1);patch([0 1 1 1-e 1-e 0+e],[0 0 1 1-e 0+e 0+e],c2);patch([0 0 1 1-e 0+e 0+e],[0 1 1 1-e 1-e 0+e],c3);plot([0 1 1 0 0],[0 0 1 1 0]);
  mux : Mux  Inputs=1
      mask Display: e = 0.06;c1 = [120 150 230]/255;c2 = ([120 150 230]+0)/383;c3 = ([120 150 230]+128)/383;patch([0 1 1 0],[0 0 1 1],c1);patch([0 1 1 1-e 1-e 0+e],[0 0 1 1-e 0+e 0+e],c2);patch([0 0 1 1-e 0+e 0+e],[0 1 1 1-e 1-e 0+e],c3);plot([0 1 1 0 0],[0 0 1 1 0]);disp('Mux')
  "pd{2,1}" : Outport
      mask Display: e = 0.06;c1 = [120 230 180]/255;c2 = ([120 230 180]+0)/(256+128);c3 = ([120 230 180]+128)/(256+128);patch([0 1 1 0],[0 0 1 1],c1);patch([0 1 1 1-e 1-e 0+e],[0 0 1 1-e 0+e 0+e],c2);patch([0 0 1 1-e 0+e 0+e],[0 1 1 1-e 1-e 0+e],c3);plot([0 1 1 0 0],[0 0 1 1 0]);
  wires:
  "p{2}"/1 -> mux/1
  mux/1 -> "pd{2,1}"/1
